simulink model "control_1"  (R2024b)
settings: Solver=FixedStepAuto  StartTime=0.0  StopTime=40.0  FixedStep=0.01  RelTol=1e-3
settings Model: Creator=Julen Beraza  LastModifiedBy=Julen Beraza

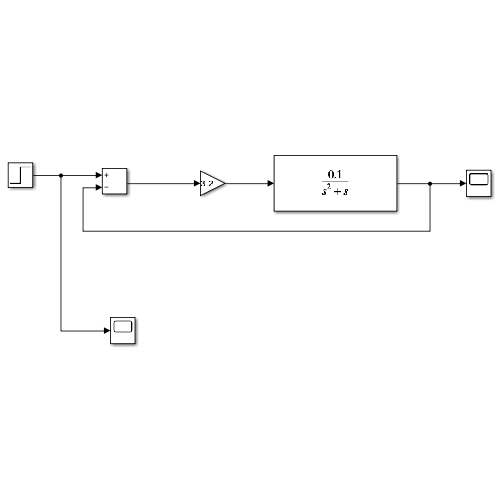
[thumbnail: Simulink's stored preview of the top-level diagram]
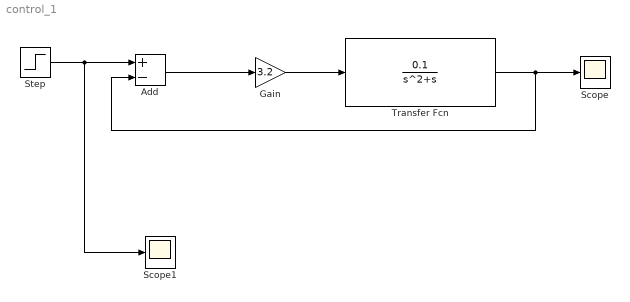
== system control_1 ==
  Add : Sum  Inputs=+-
  Gain : Gain  Gain=3.2
  Scope : Scope
  Scope1 : Scope
  Step : Step  SampleTime=0
  Transfer Fcn : TransferFcn  Numerator=[0.1]  Denominator=[1 1 0]
  wires:
  Step/1 -> Scope1/1, Add/1
  Transfer Fcn/1 -> Add/2, Scope/1
  Add/1 -> Gain/1
  Gain/1 -> Transfer Fcn/1
